simulink model "SimulinkFblock"  (R2020b)
settings: Solver=VariableStepAuto  StartTime=0.0  StopTime=10.0  RelTol=1e-3
settings Model: Creator=MikeyG  LastModifiedBy=MikeyG
settings DataIOCC: SaveFormat=Array

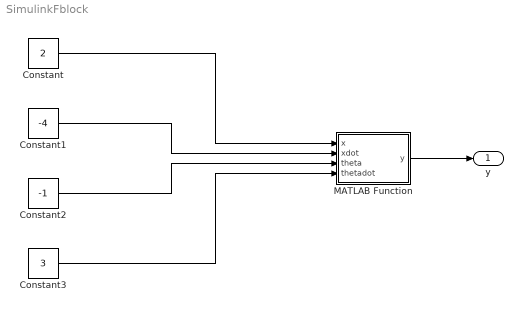
== system SimulinkFblock ==
  Constant : Constant  Value=2
  Constant1 : Constant  Value=-4
  Constant2 : Constant  Value=-1
  Constant3 : Constant  Value=3
  MATLAB Function : MATLAB Function  TreatAsAtomicUnit=on
  y : Outport  SignalName=simOut
  wires:
  Constant/1 -> MATLAB Function/1(x)
  Constant1/1 -> MATLAB Function/2(xdot)
  Constant2/1 -> MATLAB Function/3(theta)
  Constant3/1 -> MATLAB Function/4(thetadot)
  MATLAB Function/1(y) -> y/1

== matlab function SimulinkFblock/MATLAB Function ==
  data: x input; y output; xdot input; theta input; thetadot input
function y = fcn(x, xdot, theta, thetadot)

y = simFunct(x, xdot, theta, thetadot);
